simulink model "airflow"  (R2016b)
settings: Solver=VariableStepAuto  StartTime=0.0  StopTime=10  RelTol=1e-3  AbsTol=1e-3  EnableMultiTasking=on
libraries: fl_lib x17, nesl_utility x17
(part 2 of 2)

== system airflow/Subsystem2 ==
